simulink model "serial_communicator"  (R2019b)
settings: Solver=VariableStepAuto  StartTime=0.0  StopTime=10.0  RelTol=1e-3
undefined symbols (not defined in the file): Serial_Port, Standard_Devices
libraries: sldrtlib x2
settings Model: Creator=Admin  LastModifiedBy=Admin

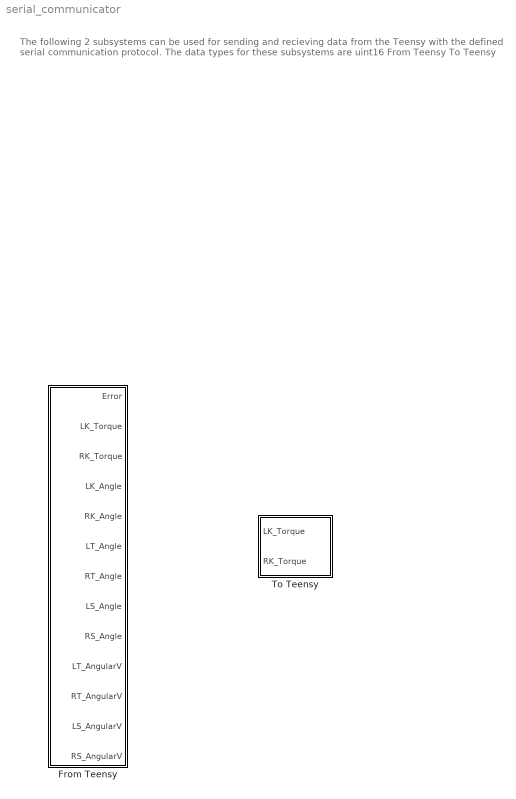
== system serial_communicator ==
  note: The following 2 subsystems can be used for sending
      | and recieving data from the Teensy with the defined serial
      | communication protocol. The data types for these subsystems
      | are uint16
      |
      | From Teensy
      |
      | To Teensy
  From Teensy : Subsystem
  To Teensy : Subsystem

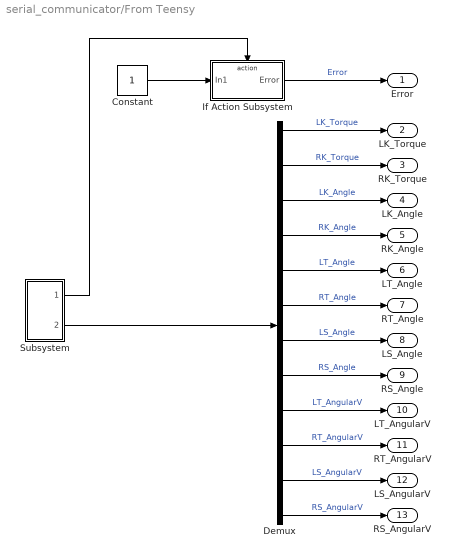
== system serial_communicator/From Teensy ==
  Constant : Constant
  Demux : Demux  Outputs=12
  If Action Subsystem : Subsystem  TreatAsAtomicUnit=on
  Subsystem : Subsystem
  Error : Outport
  LK_Torque : Outport  Port=2
  RK_Torque : Outport  Port=3
  LK_Angle : Outport  Port=4
  RK_Angle : Outport  Port=5
  LT_Angle : Outport  Port=6
  RT_Angle : Outport  Port=7
  LS_Angle : Outport  Port=8
  RS_Angle : Outport  Port=9
  LT_AngularV : Outport  Port=10
  RT_AngularV : Outport  Port=11
  LS_AngularV : Outport  Port=12
  RS_AngularV : Outport  Port=13
  wires:
  Demux/8 -> RS_Angle/1  "RS_Angle"
  Demux/9 -> LT_AngularV/1  "LT_AngularV"
  Demux/5 -> LT_Angle/1  "LT_Angle"
  Subsystem/2(Data) -> Demux/1
  Demux/3 -> LK_Angle/1  "LK_Angle"
  Constant/1 -> If Action Subsystem/1(In1)
  Demux/11 -> LS_AngularV/1  "LS_AngularV"
  Subsystem/1(Error) -> If Action Subsystem/Action
  Demux/12 -> RS_AngularV/1  "RS_AngularV"
  Demux/2 -> RK_Torque/1  "RK_Torque"
  Demux/4 -> RK_Angle/1  "RK_Angle"
  Demux/10 -> RT_AngularV/1  "RT_AngularV"
  Demux/6 -> RT_Angle/1  "RT_Angle"
  Demux/7 -> LS_Angle/1  "LS_Angle"
  Demux/1 -> LK_Torque/1  "LK_Torque"
  If Action Subsystem/1(Error) -> Error/1  "Error"

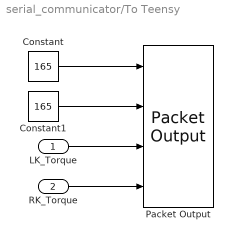
== system serial_communicator/To Teensy ==
  LK_Torque : Inport
  RK_Torque : Inport  Port=2
  Constant : Constant  Value=165
  Constant1 : Constant  Value=165
  Packet Output : sldrtlib/Packet Output  SampleTime=0.01  MaxMissedTicks=10  ShowMissedTicks=off  YieldWhenWaiting=off  DrvName=Standard_Devices/Serial_Port  DrvAddress=7  DrvOptions=[115200 8 0 0 0 0 0 0]  PacketSize=7  DataTypes={'uint8' , 'uint8' , 'uint8' , '2*uint16'}  ShowReady=off  ShowError=off  PacketID=1  ByteOrder=2  InitialValue=[]  FinalValue=[]
      settings: AttributesFormatString=Serial Port [7]  SourceProductName=Simulink Desktop Real-Time
  wires:
  Constant1/1 -> Packet Output/2
  Constant/1 -> Packet Output/1
  LK_Torque/1 -> Packet Output/3
  RK_Torque/1 -> Packet Output/4

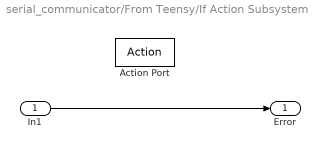
== system serial_communicator/From Teensy/If Action Subsystem ==
  In1 : Inport
  Action Port : ActionPort  ActionPortLabel=else
  Error : Outport
  wires:
  In1/1 -> Error/1

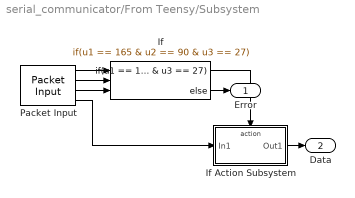
== system serial_communicator/From Teensy/Subsystem ==
  If : If  NumInputs=3  IfExpression=u1 == 165 & u2 == 90 & u3 == 27
  If Action Subsystem : Subsystem  TreatAsAtomicUnit=on
  Packet Input : sldrtlib/Packet Input  SampleTime=0.01  MaxMissedTicks=10  ShowMissedTicks=off  YieldWhenWaiting=off  DrvName=Standard_Devices/Serial_Port  DrvAddress=7  DrvOptions=[115200 8 0 0 0 0 0 0]  PacketSize=27  DataTypes={'uint8' , 'uint8' , 'uint8' , '12*uint16'}  ShowReady=off  ShowError=off  PacketID=1  ByteOrder=2  ShowTimestamp=off
      settings: AttributesFormatString=Serial Port [7]  SourceProductName=Simulink Desktop Real-Time
  Error : Outport
  Data : Outport  Port=2
  wires:
  Packet Input/4 -> If Action Subsystem/1(In1)
  If/1 -> If Action Subsystem/Action
  Packet Input/1 -> If/1
  If Action Subsystem/1(Out1) -> Data/1
  Packet Input/3 -> If/3
  If/2 -> Error/1
  Packet Input/2 -> If/2

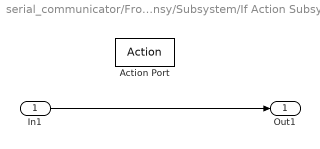
== system serial_communicator/From Teensy/Subsystem/If Action Subsystem ==
  In1 : Inport
  Action Port : ActionPort  ActionPortLabel=if(u1 == 165 & u2 == 90 & u3 == 27)
  Out1 : Outport
  wires:
  In1/1 -> Out1/1
